simulink model "quadrotor_default_2021a"  (R2021a)
settings: Solver=VariableStepAuto  StartTime=0.0  StopTime=119.35  RelTol=1e-3
InitFcn:
  | Kp_yaw = 50;
  | Kd_yaw = 0.5;
  | Kp_height = 1000;
  | Kd_height = 0.1;
  | Kp_vel = 0.15;
  | Kd_vel = 0.85;
  | Kp_attitude = 2;
  | Kd_attitude = 0.3;
  | 
  | z_des = 5;
  | 
  | sample_interval = 0.05;
  | mdl_quadrotor;
undefined symbols (not defined in the file or in its folder): rot2, x_des, y_des
libraries: roblocks x4
settings Model: Creator=SPb19  LastModifiedBy=SPb19
settings DebuggingCC: UnconnectedInputMsg=none  UnconnectedOutputMsg=none  UnconnectedLineMsg=none
settings ModelReferenceCC: EnableRefExpFcnMdlSchedulingChecks=off
settings RTWCC: Description=Generic Real-Time Target  DLArmComputeVersion=20.02.1

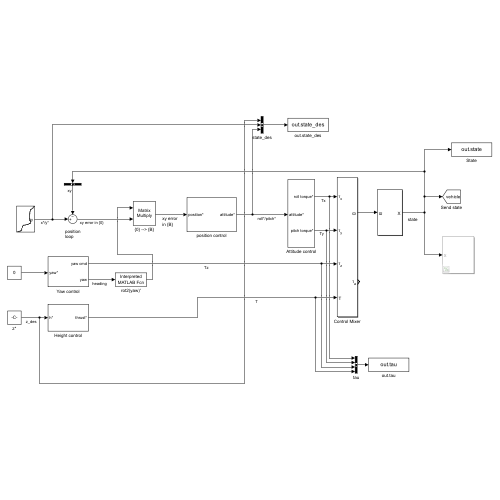
[thumbnail: Simulink's stored preview of the top-level diagram]
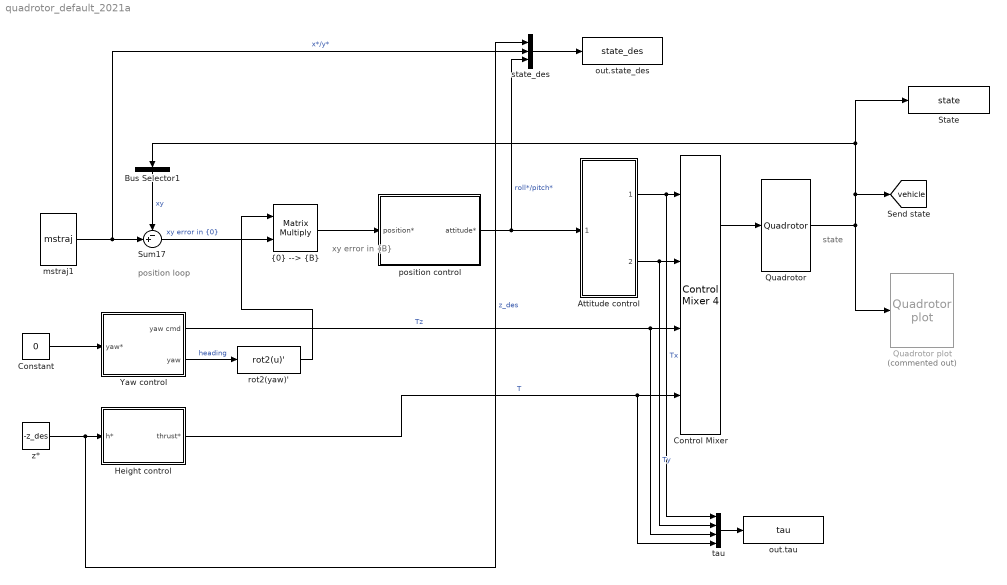
== system quadrotor_default_2021a ==
  note: state
  note: xy error
      | in {B}
  note: position
      | loop
  Attitude control : Subsystem  mask{P=Kp_attitude, D=Kd_attitude}
      mask prompts: P "Proportional gain"; D "Derivative gain"
  Bus Selector1 : BusSelector  OutputSignals=X,Y  OutputAsBus=on
  Constant : Constant  Value=0
  Control Mixer : roblocks/Vehicles/Control Mixer 4  quad=quadrotor  maxrot=1000  minrot=5
  Height control : Subsystem  mask{P=Kp_height, D=Kd_height, T0=40}
      mask prompts: P "Proportional gain"; D "Derivative gain"; T0 "Thrust feedforward"
  Quadrotor : roblocks/Vehicles/Quadrotor  quad=quadrotor  x0=[x_des(1), y_des(1) -z_des]  groundflag=on
  Quadrotor plot : roblocks/Vehicles/Quadrotor plot  Commented=on  quad=quadrotor  xydim=2  zdim=10
  State : ToWorkspace  VariableName=state  SaveFormat=Timeseries  SampleTime=-1
  Sum17 : Sum  Inputs=-+|
  Yaw control : Subsystem  mask{P=Kp_yaw, D=Kd_yaw}
      mask prompts: P "Proportional gain"; D "Derivative gain"
  mstraj1 : roblocks/Toolbox/mstraj  path=[x_des, y_des]  vaxis=[1 1]  tseg=[]  dt=sample_interval  tacc=0  setsimtime=on
  out.state_des : ToWorkspace  VariableName=state_des  SaveFormat=Timeseries  SampleTime=-1
  out.tau : ToWorkspace  VariableName=tau  SaveFormat=Timeseries  SampleTime=-1
  position control : Subsystem  mask{P=Kp_vel, D=Kd_vel}
      mask prompts: P "Proportional gain"; D "Derivative gain"
  rot2(yaw)' : MATLABFcn  MATLABFcn=rot2(u)'  OutputDimensions=[2 2]  Output1D=off
  state_des : BusCreator  Inputs=3
  tau : BusCreator  Inputs=4
  z* : Constant  Value=-z_des  SampleTime=0
  "{0} --> {B}" : Product  Multiplication=Matrix(*)  RndMeth=Zero
  tag scope: vehicle=global
  wires:
  Height control/1(thrust*) -> tau/4, Control Mixer/4  "T"
  position control/1(attitude*) -> state_des/3, Attitude control/1(attitude*)  "roll*/pitch*"
  "{0} --> {B}"/1 -> position control/1(position*)
  Yaw control/1(yaw cmd) -> tau/3, Control Mixer/3  "Tz"
  tau/1 -> out.tau/1
  Attitude control/2(pitch torque*) -> tau/2, Control Mixer/2  "Ty"
  state_des/1 -> out.state_des/1
  Sum17/1 -> "{0} --> {B}"/2  "xy error in {0}"
  Quadrotor/1 -> Quadrotor plot/1, [vehicle], State/1, Bus Selector1/1
  Control Mixer/1 -> Quadrotor/1
  Attitude control/1(roll torque*) -> tau/1, Control Mixer/1  "Tx"
  Yaw control/2(yaw) -> rot2(yaw)'/1  "heading"
  rot2(yaw)'/1 -> "{0} --> {B}"/1
  Constant/1 -> Yaw control/1(yaw*)
  z*/1 -> state_des/1, Height control/1(h*)  "z_des"
  Bus Selector1/1 -> Sum17/1  "xy"
  mstraj1/1 -> state_des/2, Sum17/2  "x*/y*"

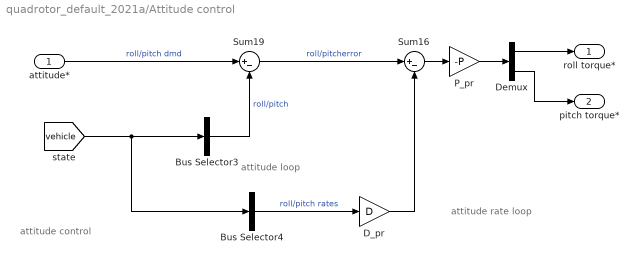
== system quadrotor_default_2021a/Attitude control ==
  note: attitude control
  note: attitude rate loop
  note: attitude loop
  attitude* : Inport
  Bus Selector3 : BusSelector  OutputSignals=roll,pitch  OutputAsBus=on
  Bus Selector4 : BusSelector  OutputSignals=droll,dpitch  OutputAsBus=on
  D_pr : Gain  Gain=D
  Demux : Demux  Outputs=2
  P_pr : Gain  Gain=-P
  Sum16 : Sum  Inputs=|+-
  Sum19 : Sum  Inputs=|+-
  roll torque* : Outport
  pitch torque* : Outport  Port=2
  wires:
  [vehicle] -> Bus Selector4/1, Bus Selector3/1
  attitude*/1 -> Sum19/1  "roll/pitch dmd"
  Bus Selector3/1 -> Sum19/2  "roll/pitch"
  Bus Selector4/1 -> D_pr/1  "roll/pitch rates"
  Sum19/1 -> Sum16/1  "roll/pitcherror"
  Sum16/1 -> P_pr/1
  P_pr/1 -> Demux/1
  D_pr/1 -> Sum16/2
  Demux/2 -> pitch torque*/1
  Demux/1 -> roll torque*/1

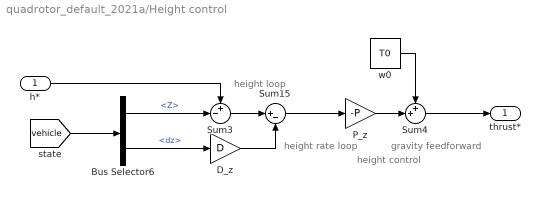
== system quadrotor_default_2021a/Height control ==
  note: height control
  note: gravity feedforward
  note: height rate
      | loop
  note: height
      | loop
  h* : Inport
  Bus Selector6 : BusSelector  OutputSignals=Z,dz
  D_z : Gain  Gain=D
  P_z : Gain  Gain=-P
  Sum15 : Sum  Inputs=|+-
  Sum3 : Sum  Inputs=+-|
  Sum4 : Sum  Inputs=++|
  w0 : Constant  Value=T0  SampleTime=0
  thrust* : Outport
  wires:
  w0/1 -> Sum4/1
  Sum15/1 -> P_z/1
  P_z/1 -> Sum4/2
  Bus Selector6/1 -> Sum3/2  "<Z>"
  h*/1 -> Sum3/1
  Sum3/1 -> Sum15/1
  Bus Selector6/2 -> D_z/1  "<dz>"
  D_z/1 -> Sum15/2
  Sum4/1 -> thrust*/1
  [vehicle] -> Bus Selector6/1

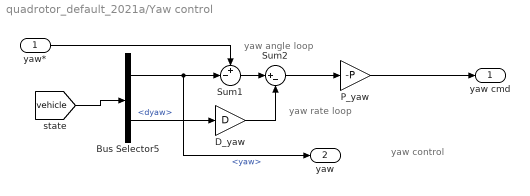
== system quadrotor_default_2021a/Yaw control ==
  note: yaw control
  note: yaw rate
      | loop
  note: yaw angle
      | loop
  yaw* : Inport
  Bus Selector5 : BusSelector  OutputSignals=yaw,dyaw
  D_yaw : Gain  Gain=D
  P_yaw : Gain  Gain=-P
  Sum1 : Sum  Inputs=+-|
  Sum2 : Sum  Inputs=|+-
  yaw cmd : Outport
  yaw : Outport  Port=2
  wires:
  [vehicle] -> Bus Selector5/1
  P_yaw/1 -> yaw cmd/1
  Bus Selector5/1 -> yaw/1, Sum1/2  "<yaw>"
  Sum2/1 -> P_yaw/1
  Bus Selector5/2 -> D_yaw/1  "<dyaw>"
  D_yaw/1 -> Sum2/2
  Sum1/1 -> Sum2/1
  yaw*/1 -> Sum1/1

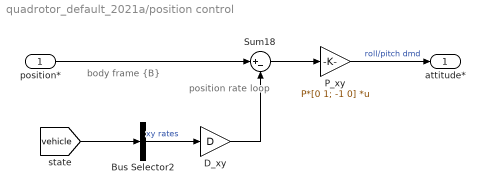
== system quadrotor_default_2021a/position control ==
  note: body frame {B}
  note: position rate
      | loop
  position* : Inport
  Bus Selector2 : BusSelector  OutputSignals=dx,dy  OutputAsBus=on
  D_xy : Gain  Gain=D
  P_xy : Gain  Gain=P*[0 1; -1 0]  Multiplication=Matrix(K*u)
  Sum18 : Sum  Inputs=|+-
  attitude* : Outport
  wires:
  Bus Selector2/1 -> D_xy/1  "xy rates"
  D_xy/1 -> Sum18/2
  Sum18/1 -> P_xy/1
  position*/1 -> Sum18/1
  [vehicle] -> Bus Selector2/1
  P_xy/1 -> attitude*/1  "roll/pitch dmd"
